simulink model "sampleModel1783"  (R2023a)
settings: Solver=VariableStepAuto  StartTime=0.0  StopTime=10.0  RelTol=1e-3
libraries: hdlsllib x3, simulink x1
settings Model: Creator=user1  LastModifiedBy=user1

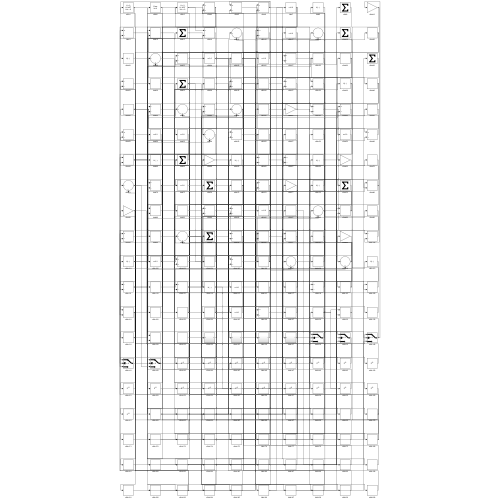
[thumbnail: Simulink's stored preview of the top-level diagram]
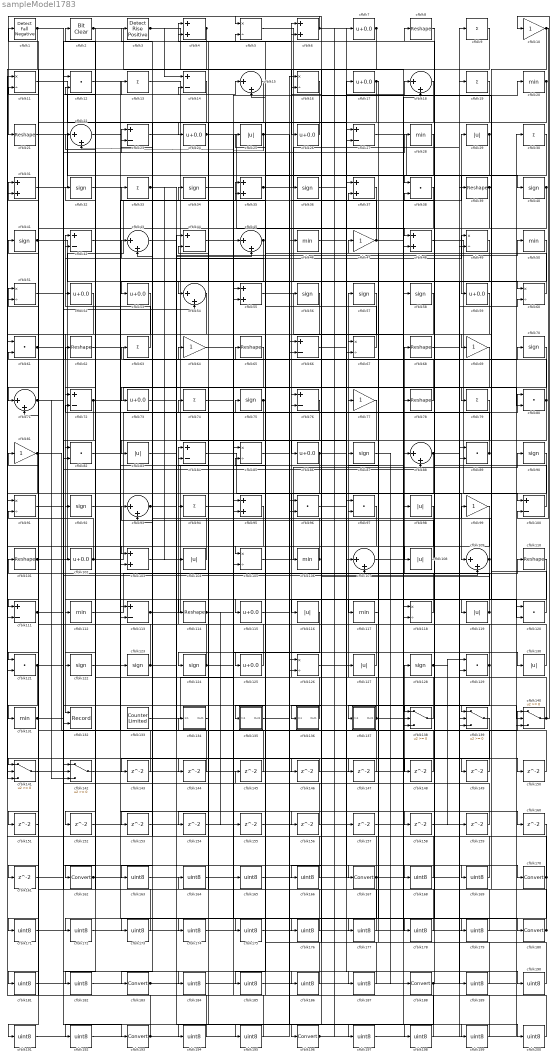
== system sampleModel1783 ==
  cfblk1 : hdlsllib/Logic and Bit Operations/Detect Fall Negative  vinit=0  OutDataTypeStr=boolean
  cfblk{10,47,64,69,77,81,99} (7 alike) : Gain
  cfblk{14,23,27,42,44,66,72,76,84,100,111,113} (12 alike) : Sum  Inputs=+-
  cfblk{8,21,39,62,65,68,78,101,110,114} (10 alike) : Reshape
  cfblk{7,17,24,26,52..53,59,73,86,102,115,125} (12 alike) : Bias  Bias=0.0  SaturateOnIntegerOverflow=off
  cfblk{4,6,31,35,37,48,55,95,103} (9 alike) : Sum
  cfblk{25,29,83,98,104,108,116,119,127,130} (10 alike) : Abs  SaturateOnIntegerOverflow=off
  cfblk{5,11,16,49,51,60,67,85,91,105,118,126} (12 alike) : Product  Inputs=*/  RndMeth=Zero  SaturateOnIntegerOverflow=on
  cfblk{20,28,46,50,106,112,117,131} (8 alike) : MinMax
  cfblk{15,18,22,43,45,54,71,88,93,107,109} (11 alike) : Sum  Inputs=|++
  cfblk{12,38,61,80,82,89,96..97,120..121,129} (11 alike) : DotProduct  OutDataTypeStr=Inherit: Inherit via internal rule
  cfblk{32,34,36,40..41,56..58,70,75,87,90,92,122..124,128} (17 alike) : Signum
  cfblk{9,13,19,30,33,63,74,79,94} (9 alike) : Sum  Inputs=+
  cfblk132 : Record  FileSettingsInternal="{\"entries\":[{\"content\":{\"excelSettings\":{\"content\":{},\"type\":\"Streamout.ExcelSettings\"}},\"type\":\"Streamout.FileSettingStorage\",\"uuid\":\"\"}],\"packageUris\":[\"http:\\/\\/schema.mathworks.com\\/mf0\\/streamout_blocks\\/R2020a\"],\"version\":\"1.0\"}"  Layout=[1 1]  SignalsInternal="{\"entries\":[{\"content\":{\"signals\":[{\"content\":{\"blockPath\":[],\"dimensions\":[1],\"domain\":\"\",\"lineColor\":\"#a2142f\",\"plots\":[1],\"port\":1,\"signalID\":3990,\"signalName\":\"XY Graph:1\"},\"type\":\"RecordBlkView.Signal\",\"uuid\":\"\"},{\"content\":{\"blockPath\":[],\"dimensions\":[1],\"domain\":\"\",\"lineColor\":\"#139fff\",\"plots\":[1],\"port\":2,\"signalID\":3993,\"signalName\":\"XY Graph:2\"},\"type\":\"RecordBlkView.Signal\",\"uuid\":\"\"}]},\"type\":\"RecordBlkView.InputSignals\",\"uuid\":\"\"}],\"packageUris\":[\"http:\\/\\/schema.mathworks.com\\/mf0\\/streamout_blocks\\/R2020a\"],\"version\":\"1.0\"}"  VisualizationBindings="{\"xyplotplugin\":{\"info\":[{\"series\":[{\"bindingParametersList\":[{\"parameter\":\"X-Axis\",\"signalID\":3990,\"signalName\":\"XY Graph:1\"},{\"parameter\":\"Y-Axis\",\"signalID\":3993,\"signalName\":\"XY Graph:2\"}],\"seriesID\":61873}],\"subplotID\":1}]}}"  CompatibilityTag=XY  st=-1
  cfblk133 : hdlsllib/Sources/Counter Limited  uplimit=7  tsamp=-1
  cfblk134 : Subsystem
      settings: LibrarySourceBlock=|
      | hdlsllib/Ports &
      | Subsystems/Subsystem
  cfblk135 : Subsystem
      settings: LibrarySourceBlock=|
      | hdlsllib/Ports &
      | Subsystems/Subsystem
  cfblk136 : Subsystem
      settings: LibrarySourceBlock=|
      | hdlsllib/Ports &
      | Subsystems/Subsystem
  cfblk137 : Subsystem
      settings: LibrarySourceBlock=|
      | hdlsllib/Ports &
      | Subsystems/Subsystem
  cfblk{138..142} (5 alike) : Switch  SaturateOnIntegerOverflow=off  InputSameDT=off
  cfblk{143..161} (19 alike) : Delay  SampleTime=1
  cfblk{162,167,170,180,183,188,193,196} (8 alike) : DataTypeConversion  SaturateOnIntegerOverflow=off  RndMeth=Floor
  cfblk{163..166,168..169,171..179,181..182,184..187,189..192,194..195,197..200} (31 alike) : DataTypeConversion  OutDataTypeStr=uint8  SaturateOnIntegerOverflow=off  RndMeth=Floor
  cfblk2 : simulink/Logic and Bit Operations/Bit Clear  iBit=0
      settings: LibrarySourceBlock=|
      | hdlsllib/Logic and Bit
      | Operations/Bit Clear
  cfblk3 : hdlsllib/Logic and Bit Operations/Detect Rise Positive  vinit=0  OutDataTypeStr=boolean
  wires:
  cfblk119/1 -> cfblk68/1, cfblk76/1
  cfblk136/1(Out1) -> cfblk6/1
  cfblk53/1 -> cfblk132/1
  cfblk62/1 -> cfblk65/1
  cfblk81/1 -> cfblk140/1, cfblk141/3
  cfblk30/1 -> cfblk196/1
  cfblk45/1 -> cfblk53/1, cfblk42/2
  cfblk63/1 -> cfblk42/1
  cfblk31/1 -> cfblk13/1
  cfblk24/1 -> cfblk48/1, cfblk140/2, cfblk130/1
  cfblk120/1 -> cfblk21/1
  cfblk102/1 -> cfblk75/1, cfblk41/1
  cfblk48/1 -> cfblk100/1
  cfblk118/1 -> cfblk101/1
  cfblk66/1 -> cfblk170/1
  cfblk60/1 -> cfblk33/1
  cfblk108/1 -> cfblk93/1
  cfblk138/1 -> cfblk57/1
  cfblk21/1 -> cfblk38/1
  cfblk90/1 -> cfblk103/1
  cfblk127/1 -> cfblk84/1
  cfblk101/1 -> cfblk29/1, cfblk6/2, cfblk181/1
  cfblk5/1 -> cfblk60/1
  cfblk20/1 -> cfblk72/1, cfblk54/1
  cfblk69/1 -> cfblk124/1
  cfblk23/1 -> cfblk127/1
  cfblk92/1 -> cfblk35/1
  cfblk91/1 -> cfblk193/1
  cfblk123/1 -> cfblk52/1, cfblk187/1
  cfblk29/1 -> cfblk105/1, cfblk108/1
  cfblk27/1 -> cfblk59/1
  cfblk125/1 -> cfblk74/1
  cfblk72/1 -> cfblk79/1, cfblk82/2
  cfblk112/1 -> cfblk110/1
  cfblk111/1 -> cfblk88/2, cfblk184/1
  cfblk3/1 -> cfblk14/1, cfblk107/2
  cfblk37/1 -> cfblk125/1
  cfblk128/1 -> cfblk129/1, cfblk159/1
  cfblk114/1 -> cfblk129/2, cfblk155/1
  cfblk84/1 -> cfblk109/1
  cfblk28/1 -> cfblk116/1
  cfblk13/1 -> cfblk40/1
  cfblk104/1 -> cfblk62/1
  cfblk130/1 -> cfblk2/1
  cfblk103/1 -> cfblk46/1
  cfblk86/1 -> cfblk17/1, cfblk161/1
  cfblk6/1 -> cfblk37/1, cfblk5/1
  cfblk113/1 -> cfblk55/1, cfblk49/1
  cfblk133/1 -> cfblk105/2
  cfblk9/1 -> cfblk136/1(In1)
  cfblk19/1 -> cfblk183/1
  cfblk55/1 -> cfblk118/2
  cfblk79/1 -> cfblk114/1
  cfblk109/1 -> cfblk112/1, cfblk78/1, cfblk44/2, cfblk67/1
  cfblk121/1 -> cfblk131/1, cfblk23/2
  cfblk43/1 -> cfblk167/1
  cfblk11/1 -> cfblk27/2
  cfblk100/1 -> cfblk4/1
  cfblk7/1 -> cfblk26/1, cfblk142/2, cfblk82/1
  cfblk117/1 -> cfblk77/1
  cfblk124/1 -> cfblk139/1, cfblk51/1, cfblk76/2
  cfblk134/1(Out1) -> cfblk94/1
  cfblk40/1 -> cfblk67/2, cfblk191/1
  cfblk33/1 -> cfblk104/1, cfblk147/1
  cfblk78/1 -> cfblk31/1
  cfblk65/1 -> cfblk73/1
  cfblk18/1 -> cfblk135/1(In1)
  cfblk71/1 -> cfblk15/1, cfblk142/3
  cfblk35/1 -> cfblk9/1, cfblk149/1
  cfblk89/1 -> cfblk32/1, cfblk56/1
  cfblk131/1 -> cfblk31/2, cfblk54/2
  cfblk10/1 -> cfblk100/2, cfblk69/1
  cfblk49/1 -> cfblk83/1
  cfblk51/1 -> cfblk109/2
  cfblk32/1 -> cfblk123/1
  cfblk59/1 -> cfblk111/1
  cfblk57/1 -> cfblk141/2
  cfblk97/1 -> cfblk121/1
  cfblk54/1 -> cfblk132/2
  cfblk83/1 -> cfblk70/1
  cfblk73/1 -> cfblk50/1
  cfblk137/1(Out1) -> cfblk22/1, cfblk18/2
  cfblk140/1 -> cfblk10/1, cfblk5/2
  cfblk82/1 -> cfblk34/1
  cfblk96/1 -> cfblk180/1
  cfblk135/1(Out1) -> cfblk80/1
  cfblk75/1 -> cfblk113/2, cfblk115/1
  cfblk87/1 -> cfblk188/1
  cfblk94/1 -> cfblk20/1
  cfblk41/1 -> cfblk103/2, cfblk139/2
  cfblk142/1 -> cfblk128/1
  cfblk26/1 -> cfblk24/1
  cfblk61/1 -> cfblk138/1, cfblk28/1, cfblk14/2
  cfblk129/1 -> cfblk137/1(In1), cfblk4/2
  cfblk15/1 -> cfblk92/1
  cfblk67/1 -> cfblk15/2
  cfblk44/1 -> cfblk45/1
  cfblk46/1 -> cfblk18/1
  cfblk14/1 -> cfblk71/1
  cfblk122/1 -> cfblk88/1
  cfblk88/1 -> cfblk60/2, cfblk106/1
  cfblk56/1 -> cfblk122/1
  cfblk2/1 -> cfblk48/2, cfblk182/1
  cfblk80/1 -> cfblk23/1, cfblk143/1
  cfblk115/1 -> cfblk37/2
  cfblk25/1 -> cfblk22/2, cfblk120/2, cfblk80/2, cfblk158/1
  cfblk95/1 -> cfblk162/1
  cfblk47/1 -> cfblk36/1, cfblk200/1
  cfblk98/1 -> cfblk121/2
  cfblk1/1 -> cfblk111/2, cfblk168/1
  cfblk39/1 -> cfblk86/1, cfblk119/1
  cfblk106/1 -> cfblk63/1, cfblk3/1
  cfblk93/1 -> cfblk45/2, cfblk197/1, cfblk199/1
  cfblk4/1 -> cfblk151/1, cfblk152/1
  cfblk105/1 -> cfblk90/1
  cfblk17/1 -> cfblk102/1, cfblk117/1
  cfblk143/1 -> cfblk1/1
  cfblk110/1 -> cfblk144/1
  cfblk144/1 -> cfblk113/1
  cfblk145/1 -> cfblk61/2
  cfblk74/1 -> cfblk146/1
  cfblk146/1 -> cfblk141/1
  cfblk147/1 -> cfblk35/2
  cfblk50/1 -> cfblk148/1
  cfblk148/1 -> cfblk84/2
  cfblk149/1 -> cfblk138/2
  cfblk42/1 -> cfblk150/1
  cfblk150/1 -> cfblk44/1
  cfblk151/1 -> cfblk11/2
  cfblk152/1 -> cfblk138/3
  cfblk76/1 -> cfblk153/1
  cfblk153/1 -> cfblk93/2
  cfblk99/1 -> cfblk154/1
  cfblk154/1 -> cfblk55/2
  cfblk155/1 -> cfblk27/1
  cfblk22/1 -> cfblk156/1
  cfblk156/1 -> cfblk72/2
  cfblk36/1 -> cfblk157/1
  cfblk157/1 -> cfblk118/1
  cfblk158/1 -> cfblk89/2
  cfblk159/1 -> cfblk142/1
  cfblk107/1 -> cfblk160/1
  cfblk162/1 -> cfblk49/2, cfblk107/1
  cfblk77/1 -> cfblk163/1
  cfblk163/1 -> cfblk95/1
  cfblk160/1 -> cfblk164/1
  cfblk164/1 -> cfblk95/2
  cfblk64/1 -> cfblk165/1
  cfblk165/1 -> cfblk97/1
  cfblk38/1 -> cfblk166/1
  cfblk166/1 -> cfblk64/1
  cfblk167/1 -> cfblk97/2, cfblk11/1, cfblk172/1
  cfblk168/1 -> cfblk43/1
  cfblk161/1 -> cfblk169/1
  cfblk169/1 -> cfblk43/2
  cfblk170/1 -> cfblk51/2, cfblk38/2, cfblk194/1
  cfblk52/1 -> cfblk171/1
  cfblk171/1 -> cfblk66/1
  cfblk172/1 -> cfblk66/2
  cfblk58/1 -> cfblk173/1
  cfblk173/1 -> cfblk81/1
  cfblk116/1 -> cfblk174/1
  cfblk174/1 -> cfblk58/1
  cfblk12/1 -> cfblk175/1
  cfblk175/1 -> cfblk120/1
  cfblk139/1 -> cfblk176/1
  cfblk176/1 -> cfblk12/1
  cfblk70/1 -> cfblk177/1
  cfblk177/1 -> cfblk12/2
  cfblk8/1 -> cfblk178/1
  cfblk178/1 -> cfblk47/1
  cfblk34/1 -> cfblk179/1
  cfblk179/1 -> cfblk8/1
  cfblk180/1 -> cfblk134/1(In1), cfblk99/1
  cfblk181/1 -> cfblk96/1
  cfblk182/1 -> cfblk96/2
  cfblk183/1 -> cfblk89/1, cfblk195/1
  cfblk184/1 -> cfblk19/1
  cfblk16/1 -> cfblk185/1
  cfblk185/1 -> cfblk39/1
  cfblk141/1 -> cfblk186/1
  cfblk186/1 -> cfblk16/1
  cfblk187/1 -> cfblk16/2
  cfblk188/1 -> cfblk140/3, cfblk98/1, cfblk192/1
  cfblk68/1 -> cfblk189/1
  cfblk189/1 -> cfblk87/1
  cfblk126/1 -> cfblk190/1
  cfblk190/1 -> cfblk145/1
  cfblk191/1 -> cfblk126/1
  cfblk192/1 -> cfblk126/2
  cfblk193/1 -> cfblk71/2, cfblk61/1
  cfblk194/1 -> cfblk91/1
  cfblk195/1 -> cfblk91/2
  cfblk196/1 -> cfblk139/3, cfblk7/1
  cfblk197/1 -> cfblk30/1
  cfblk85/1 -> cfblk198/1
  cfblk198/1 -> cfblk25/1
  cfblk199/1 -> cfblk85/1
  cfblk200/1 -> cfblk85/2

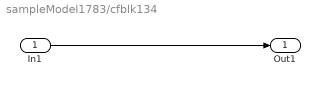
== system sampleModel1783/cfblk134 ==
  In1 : Inport
  Out1 : Outport
  wires:
  In1/1 -> Out1/1

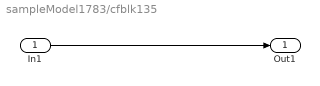
== system sampleModel1783/cfblk135 ==
  In1 : Inport
  Out1 : Outport
  wires:
  In1/1 -> Out1/1

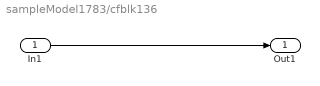
== system sampleModel1783/cfblk136 ==
  In1 : Inport
  Out1 : Outport
  wires:
  In1/1 -> Out1/1

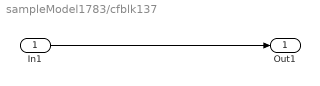
== system sampleModel1783/cfblk137 ==
  In1 : Inport
  Out1 : Outport
  wires:
  In1/1 -> Out1/1
